simulink model "Exp_100_StepTest"  (R2016a)
settings: Solver=ode45  StartTime=0.0  StopTime=700  RelTol=1e-3
StartFcn:
  | clear all
libraries: realtime_pacer_lib x1
settings Model: Creator=johnh  LastModifiedBy=tiago
settings DataIOCC: SaveFormat=StructureWithTime
settings HardwareCC: ProdWordSize=32  ProdHWDeviceType=Specified
settings ConfigComp: CovModelRefEnable=Off

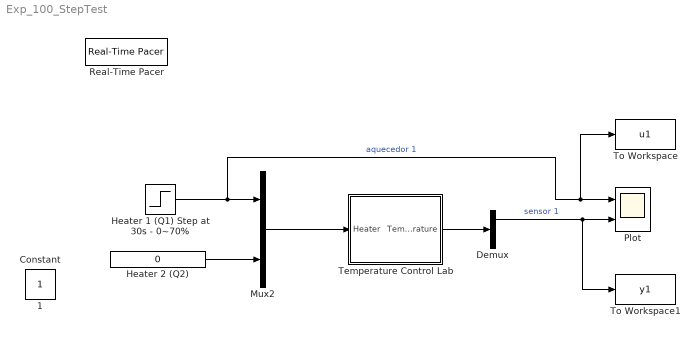
== system Exp_100_StepTest ==
  Demux : Demux  Outputs=2
  Heater 1 (Q1) Step at 30s - 0~70% : Step  Time=30  After=70  SampleTime=0
  Heater 2 (Q2) : Constant  Value=0
  Mux2 : Mux  Inputs=2
  Plot : Scope  NumInputPorts=2
  Real-Time Pacer : realtime_pacer_lib/Real-Time Pacer  simTimePerRealTime=1
  Temperature Control Lab : Subsystem
      mask Display: image('tclab.png');
  To Workspace : ToWorkspace  VariableName=u1  SaveFormat=Timeseries  SampleTime=-1
  To Workspace1 : ToWorkspace  VariableName=y1  SaveFormat=Timeseries  SampleTime=-1
  1 : Constant  IOType=siggen
  Constant : Constant  IOType=siggen
  wires:
  Heater 2 (Q2)/1 -> Mux2/2
  Mux2/1 -> Temperature Control Lab/1(Heater)
  Temperature Control Lab/1(Temperature) -> Demux/1
  Heater 1 (Q1) Step at 30s - 0~70%/1 -> To Workspace/1, Plot/1, Mux2/1  "aquecedor 1"
  Demux/1 -> To Workspace1/1, Plot/2  "sensor 1"

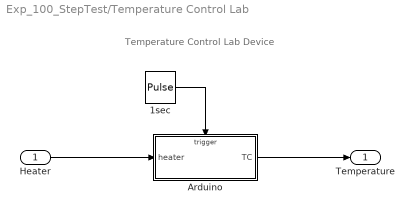
== system Exp_100_StepTest/Temperature Control Lab ==
  note: Temperature Control Lab Device
  Heater : Inport
  1sec : DiscretePulseGenerator  PulseType=Time based  Period=1  PulseWidth=50
  Arduino : Subsystem  TreatAsAtomicUnit=on
  Temperature : Outport
  wires:
  1sec/1 -> Arduino/Trigger
  Arduino/1(TC) -> Temperature/1
  Heater/1 -> Arduino/1(heater)

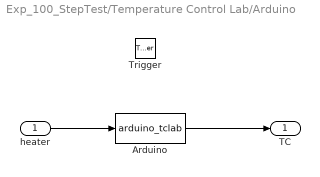
== system Exp_100_StepTest/Temperature Control Lab/Arduino ==
  heater : Inport  LatchByDelayingOutsideSignal=on
  Trigger : TriggerPort  VariantControl=Variant
  Arduino : MATLABFcn  MATLABFcn=arduino_tclab
  TC : Outport  InitialOutput=[23 23]
  wires:
  heater/1 -> Arduino/1
  Arduino/1 -> TC/1
